simulink model "CS_project_02_r2018b"  (R2018b)
settings: Solver=ode45  StartTime=0.0  StopTime=0.1  RelTol=1e-3
libraries: simulink x1
settings Model: Creator=yasho  LastModifiedBy=shubh

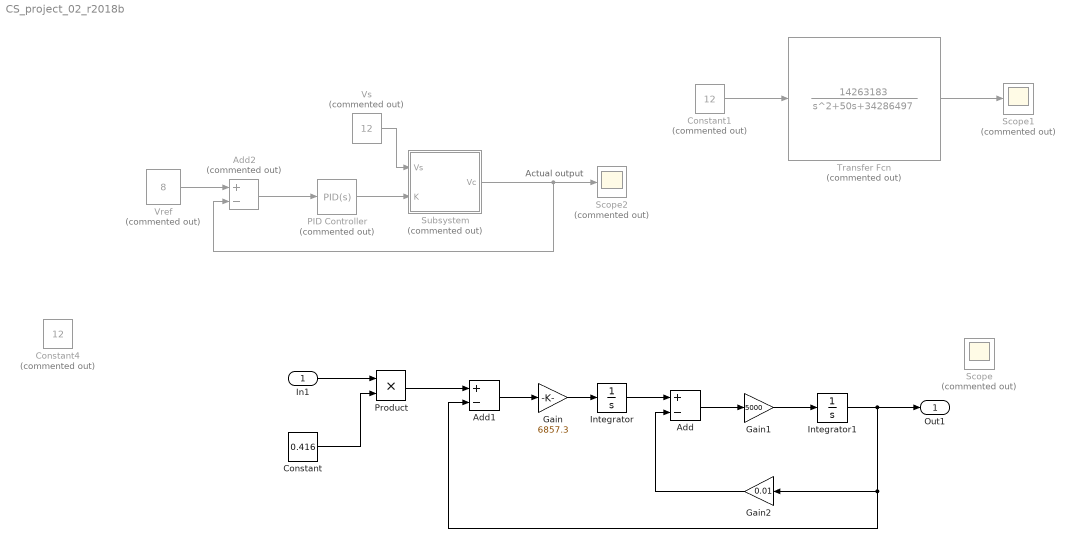
== system CS_project_02_r2018b ==
  note: Actual output
  In1 : Inport
  Add : Sum  Inputs=+-
  Add1 : Sum  Inputs=+-
  Add2 : Sum  Commented=on  Inputs=+-
  Constant : Constant  Value=0.416
  Constant1 : Constant  Commented=on  Value=12
  Constant4 : Constant  Commented=on  Value=12
  Gain : Gain  Gain=6857.3
  Gain1 : Gain  Gain=5000
  Gain2 : Gain  Gain=0.01
  Integrator : Integrator
  Integrator1 : Integrator
  PID Controller : simulink/Continuous/PID Controller  Commented=on  Controller=PID  Form=Parallel  TimeDomain=Continuous-time  SampleTime=-1  IntegratorMethod=Forward Euler  FilterMethod=Forward Euler  ControllerParametersSource=internal  P=2.7770310187959  I=7033.65699351539  D=0.000223614544652275  UseFilter=on  N=10623866.1667962  TunerSelectOption=Transfer Function Based (PID Tuner App)  InitialConditionSource=internal  InitialConditionForIntegrator=0  InitialConditionForFilter=0  DifferentiatorICPrevScaledInput=0  ExternalReset=none  TrackingMode=off  Kt=1  LimitOutput=off  UpperSaturationLimit=inf  LowerSaturationLimit=-inf  LinearizeAsGain=on  AntiWindupMode=none  Kb=1  POutMin=[]  POutMax=[]  IOutMin=[]  IOutMax=[]  DOutMin=[]  DOutMax=[]  NOutMin=[]  NOutMax=[]  SumOutMin=[]  SumOutMax=[]  SaturationOutMin=[]  SaturationOutMax=[]  PParamMin=[]  PParamMax=[]  IParamMin=[]  IParamMax=[]  DParamMin=[]  DParamMax=[]  NParamMin=[]  NParamMax=[]  KbParamMin=[]  KbParamMax=[]  KtParamMin=[]  KtParamMax=[]  KbOutMin=[]  KbOutMax=[]  KtOutMin=[]  KtOutMax=[]  IntegratorOutMin=[]  IntegratorOutMax=[]  FilterOutMin=[]  FilterOutMax=[]  SumI1OutMin=[]  SumI1OutMax=[]  SumI2OutMin=[]  SumI2OutMax=[]  SumI3OutMin=[]  SumI3OutMax=[]  SumI4OutMin=[]  SumI4OutMax=[]  SumDOutMin=[]  SumDOutMax=[]  DifferentiatorOutMin=[]  DifferentiatorOutMax=[]  FilterDiffOutCoefMin=[]  FilterDiffOutCoefMax=[]  ReciprocalOutMin=[]  ReciprocalOutMax=[]  SumDenOutMin=[]  SumDenOutMax=[]  SumNumOutMin=[]  SumNumOutMax=[]  DivideOutMin=[]  DivideOutMax=[]  IntegratorContinuousStateAttributes=''  IntegratorStateMustResolveToSignalObject=off  IntegratorRTWStateStorageClass=Auto  FilterContinuousStateAttributes=''  FilterStateMustResolveToSignalObject=off  FilterRTWStateStorageClass=Auto  ParallelPVariant=InternalParameters  IdealPVariant=Disabled  IVariant=InternalParameters  DVariant=InternalParameters  IntegratorVariant=Continuous  SatVariant=Disabled  AWVariant=Passthrough  PCopyVariant=Disabled  TRVariant=Disabled  FdbkBlocksVariant=Forward  IdealPFdbkVariant=Disabled  SatFdbkVariant=Disabled  DerivativeFilterVariant=ContFilter  NVariant=InternalParameters  NCopyVariant=Disabled  FilterICVariant=InternalICsFilter  IntegratorICVariant=InternalICs  ExternalResetVariant=Disabled  TRSumVariant=Passthrough  SumFdbkVariant=Disabled  SumVariant=Sum_PID
  Product : Product
  Scope : Scope  Commented=on
  Scope1 : Scope  Commented=on
  Scope2 : Scope  Commented=on
  Subsystem : Subsystem  Commented=on
  Transfer Fcn : TransferFcn  Commented=on  Numerator=[14263183]  Denominator=[1 50 34286497]
  Vref : Constant  Commented=on  Value=8
  Vs : Constant  Commented=on  Value=12
  Out1 : Outport
  wires:
  Add2/1 -> PID Controller/1
  Vref/1 -> Add2/1
  Constant1/1 -> Transfer Fcn/1
  Transfer Fcn/1 -> Scope1/1
  Subsystem/1(Vc) -> Add2/2, Scope2/1
  PID Controller/1 -> Subsystem/2(K)
  Vs/1 -> Subsystem/1(Vs)
  Gain/1 -> Integrator/1
  Product/1 -> Add1/1
  Add1/1 -> Gain/1
  In1/1 -> Product/1
  Gain2/1 -> Add/2
  Gain1/1 -> Integrator1/1
  Add/1 -> Gain1/1
  Constant/1 -> Product/2
  Integrator1/1 -> Out1/1, Gain2/1, Add1/2
  Integrator/1 -> Add/1

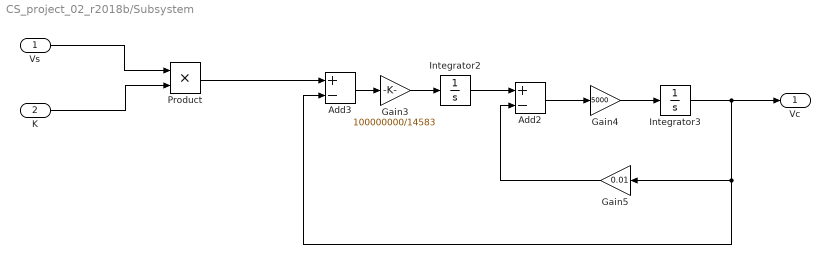
== system CS_project_02_r2018b/Subsystem ==
  Vs : Inport
  K : Inport  Port=2
  Add2 : Sum  Inputs=+-
  Add3 : Sum  Inputs=+-
  Gain3 : Gain  Gain=100000000/14583
  Gain4 : Gain  Gain=5000
  Gain5 : Gain  Gain=0.01
  Integrator2 : Integrator
  Integrator3 : Integrator
  Product : Product
  Vc : Outport  VectorParamsAs1DForOutWhenUnconnected=on
  wires:
  Integrator2/1 -> Add2/1
  Gain4/1 -> Integrator3/1
  Integrator3/1 -> Vc/1, Add3/2, Gain5/1
  Add3/1 -> Gain3/1
  Gain3/1 -> Integrator2/1
  Add2/1 -> Gain4/1
  Gain5/1 -> Add2/2
  Product/1 -> Add3/1
  Vs/1 -> Product/1
  K/1 -> Product/2
